simulink model "SubsysUnchanged"  (R2023b)
settings: Solver=VariableStepAuto  StartTime=0.0  StopTime=10.0  RelTol=1e-3
settings Model: Creator=neham  LastModifiedBy=neham

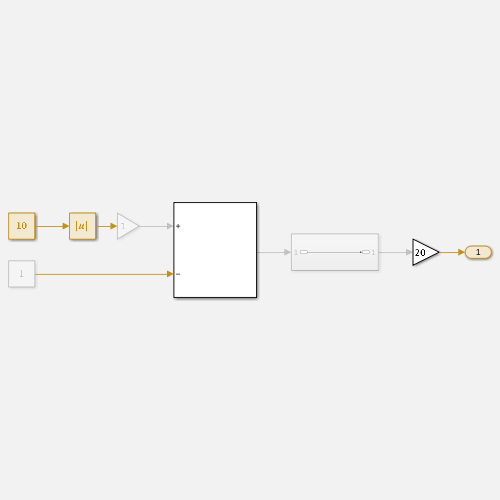
[thumbnail: Simulink's stored preview of the top-level diagram]
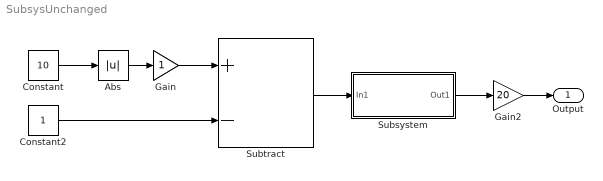
== system SubsysUnchanged ==
  Abs : Abs  SaturateOnIntegerOverflow=off
  Constant : Constant  Value=10
  Constant2 : Constant
  Gain : Gain
  Gain2 : Gain  Gain=20
  Subsystem : Subsystem
  Subtract : Sum  Inputs=+-
  Output : Outport
  wires:
  Gain/1 -> Subtract/1
  Subsystem/1(Out1) -> Gain2/1
  Constant2/1 -> Subtract/2
  Gain2/1 -> Output/1
  Subtract/1 -> Subsystem/1(In1)
  Abs/1 -> Gain/1
  Constant/1 -> Abs/1

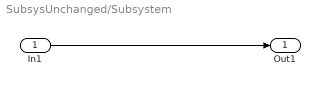
== system SubsysUnchanged/Subsystem ==
  In1 : Inport
  Out1 : Outport
  wires:
  In1/1 -> Out1/1
